simulink model "Adaptive_Distributed_Observer"  (R2016b)
settings: Solver=ode23t  StartTime=0.0  StopTime=5  RelTol=1e-3
values from neighbouring files (symbols this model uses):
  E = zeros(2,4)    [Init_ADO.m]
  F = -R    [Init_ADO.m]
  mu = 100    [Init_ADO.m]
  Mu_n = 100000    [Init_ADO.m]
  Mu_S = 10    [Init_ADO.m]
  P = [-2, -6]    [Init_ADO.m]
  R = [1 0 0 0]    [Init_ADO.m]
  S = [0 w1 0 0;-w1 0 0 0;0 0 0 w2;0 0 -w2 0]    [Init_ADO.m]
  S0 = zeros(4,4)    [Init_ADO.m]
  Z0 = ones(3*n,1)    [Init_ADO.m]
settings Model: Creator=Niels  LastModifiedBy=Niels
settings SolverCC: ZeroCrossAlgorithm=Adaptive

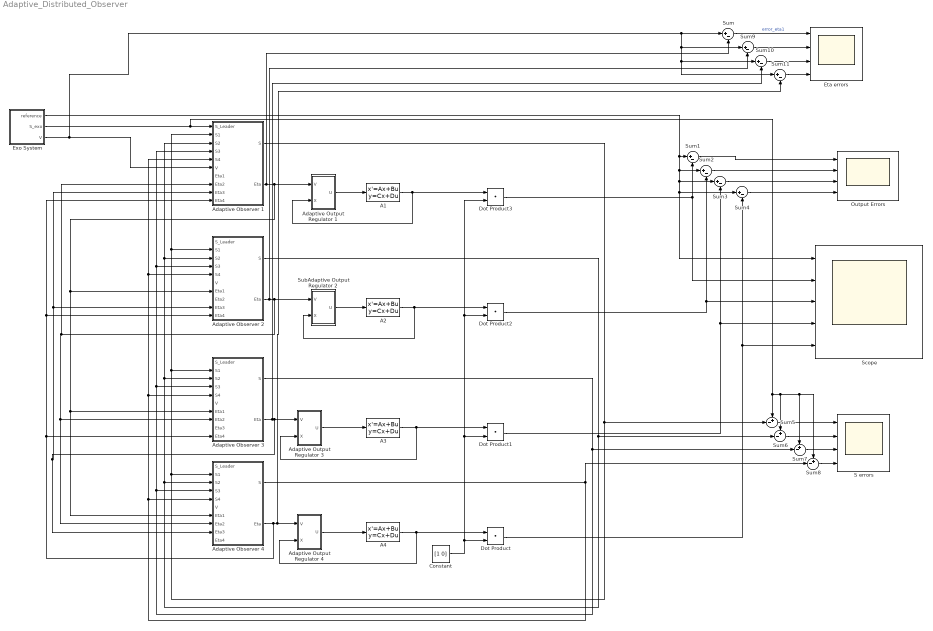
== system Adaptive_Distributed_Observer ==
  A1 : StateSpace  A=[-10 1;-24 0]  B=[2;3]  C=[1 0;0 1]  D=[0;0]  X0=0
  A2 : StateSpace  A=[-12 1;-11 0]  B=[2;1]  C=[1 0; 0 1]  D=[0;0]  X0=0
  A3 : StateSpace  A=[3 1;-1 0]  B=[1;1]  C=[1 0;0 1]  D=[0;0]  X0=0
  A4 : StateSpace  A=[2 1; -2 0]  B=[3;1]  C=[1 0;0 1]  D=[0 ;0]  X0=0
  Adaptive Observer 1 : Subsystem
  Adaptive Observer 2 : Subsystem
  Adaptive Observer 3 : Subsystem
  Adaptive Observer 4 : Subsystem
  Adaptive Output Regulator 1 : Subsystem
  Adaptive Output Regulator 3 : Subsystem
  Adaptive Output Regulator 4 : Subsystem
  Constant : Constant  Value=[1 0]
  Dot Product{,1..3} (4 alike) : DotProduct  InputSameDT=on  OutDataTypeStr=Inherit: Inherit via internal rule
  Eta errors : Scope  NumInputPorts=4
  Exo System : Subsystem
  Output Errors : Scope  NumInputPorts=4
  S errors : Scope  NumInputPorts=4
  Scope : Scope  NumInputPorts=5
  SubAdaptive Output Regulator 2 : Subsystem
  Sum{,1..4,9..11} (8 alike) : Sum  Inputs=|+-
  Sum{5..8} (4 alike) : Sum  Inputs=+-|
  wires:
  SubAdaptive Output Regulator 2/1(U) -> A2/1
  A4/1 -> Dot Product/1, Adaptive Output Regulator 4/2(X)
  A3/1 -> Dot Product1/1, Adaptive Output Regulator 3/2(X)
  Adaptive Observer 2/2(Eta) -> Sum9/2, SubAdaptive Output Regulator 2/1(V), Adaptive Observer 1/8(Eta2), Adaptive Observer 4/8(Eta2), Adaptive Observer 3/8(Eta2)
  Adaptive Observer 3/2(Eta) -> Adaptive Output Regulator 3/1(V), Adaptive Observer 1/9(Eta3), Adaptive Observer 2/9(Eta3), Adaptive Observer 4/9(Eta3), Sum10/2
  Adaptive Observer 4/2(Eta) -> Adaptive Output Regulator 4/1(V), Sum11/2, Adaptive Observer 1/10(Eta4), Adaptive Observer 2/10(Eta4), Adaptive Observer 3/10(Eta4)
  Exo System/3(V) -> Sum11/1, Sum10/1, Sum9/1, Sum/1, Adaptive Observer 1/6(V)
  Adaptive Observer 1/1(S) -> Sum5/2, Adaptive Observer 1/2("S1 "), Adaptive Observer 2/2("S1 "), Adaptive Observer 3/2("S1 "), Adaptive Observer 4/2("S1 ")
  Adaptive Observer 2/1(S) -> Adaptive Observer 1/3(S2), Adaptive Observer 2/3(S2), Adaptive Observer 3/3(S2), Adaptive Observer 4/3(S2), Sum6/2
  Adaptive Observer 3/1(S) -> Sum7/2, Adaptive Observer 1/4(S3), Adaptive Observer 2/4(S3), Adaptive Observer 3/4(S3), Adaptive Observer 4/4(S3)
  Adaptive Observer 4/1(S) -> Sum8/2, Adaptive Observer 1/5(S4), Adaptive Observer 2/5(S4), Adaptive Observer 3/5(S4), Adaptive Observer 4/5(S4)
  Adaptive Observer 1/2(Eta) -> Adaptive Output Regulator 1/1(V), Adaptive Observer 2/7(Eta1), Adaptive Observer 3/7(Eta1), Adaptive Observer 4/7(Eta1), Sum/2
  Exo System/1(reference) -> Scope/1, Sum4/1, Sum3/1, Sum2/1, Sum1/1
  A1/1 -> Dot Product3/1, Adaptive Output Regulator 1/2(X)
  Exo System/2("S_exo ") -> Sum8/1, Sum7/1, Sum6/1, Sum5/1, Adaptive Observer 1/1(S_Leader)
  Adaptive Output Regulator 1/1(U) -> A1/1
  Adaptive Output Regulator 3/1(U) -> A3/1
  Adaptive Output Regulator 4/1(U) -> A4/1
  Sum/1 -> Eta errors/1  "error_eta1"
  Sum1/1 -> Output Errors/1
  Sum2/1 -> Output Errors/2
  Sum3/1 -> Output Errors/3
  Sum4/1 -> Output Errors/4
  Sum8/1 -> S errors/4
  Sum7/1 -> S errors/3
  Sum5/1 -> S errors/1
  Sum6/1 -> S errors/2
  Sum9/1 -> Eta errors/2
  Sum10/1 -> Eta errors/3
  Sum11/1 -> Eta errors/4
  A2/1 -> Dot Product2/1, SubAdaptive Output Regulator 2/2(X)
  Dot Product/1 -> Scope/5, Sum4/2
  Dot Product1/1 -> Scope/4, Sum3/2
  Dot Product2/1 -> Scope/3, Sum2/2
  Dot Product3/1 -> Scope/2, Sum1/2
  Constant/1 -> Dot Product/2, Dot Product1/2, Dot Product2/2, Dot Product3/2

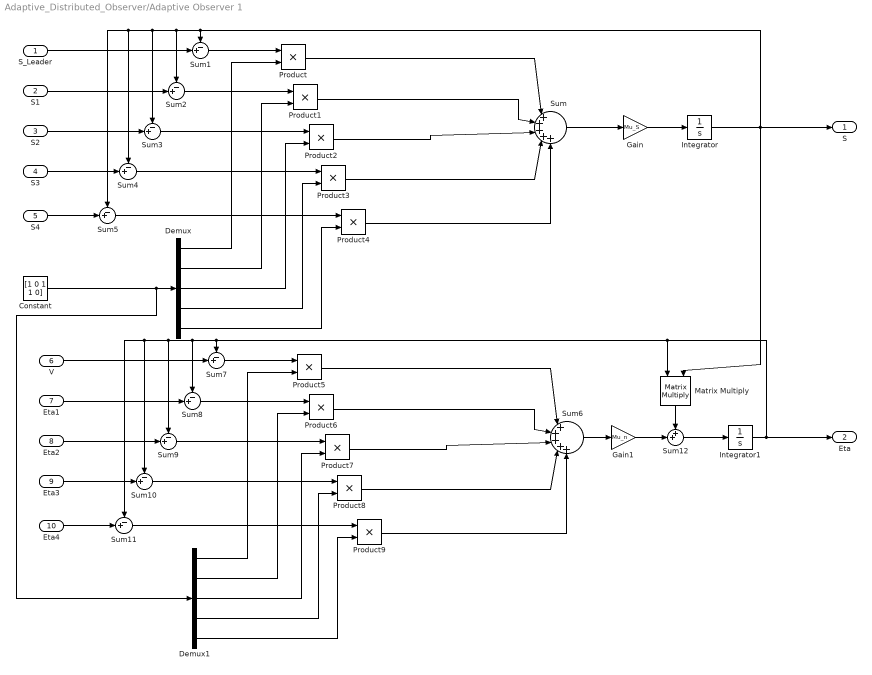
== system Adaptive_Distributed_Observer/Adaptive Observer 1 ==
  S_Leader : Inport
  "S1 " : Inport  Port=2
  S2 : Inport  Port=3
  S3 : Inport  Port=4
  S4 : Inport  Port=5
  V : Inport  Port=6
  Eta1 : Inport  Port=7
  Eta2 : Inport  Port=8
  Eta3 : Inport  Port=9
  Eta4 : Inport  Port=10
  Constant : Constant  Value=[1 0 1 1 0]
  Demux : Demux  Outputs=5
  Demux1 : Demux  Outputs=5
  Gain : Gain  Gain=Mu_S
  Gain1 : Gain  Gain=Mu_n
  Integrator : Integrator  InitialCondition=S0
  Integrator1 : Integrator
  Matrix Multiply : Product  Multiplication=Matrix(*)
  Product{,1..9} (10 alike) : Product
  Sum : Sum  Inputs=|+++++
  Sum{1..5,7..11} (10 alike) : Sum  Inputs=-+|
  Sum12 : Sum  Inputs=++|
  Sum6 : Sum  Inputs=|+++++
  S : Outport
  Eta : Outport  Port=2
  wires:
  Demux/1 -> Product/2
  Demux/2 -> Product1/2
  Demux/3 -> Product2/2
  Demux/4 -> Product3/2
  Demux/5 -> Product4/2
  Product2/1 -> Sum/3
  Product1/1 -> Sum/2
  Product/1 -> Sum/1
  Product4/1 -> Sum/5
  Product3/1 -> Sum/4
  Sum/1 -> Gain/1
  Gain/1 -> Integrator/1
  Sum1/1 -> Product/1
  S_Leader/1 -> Sum1/2
  "S1 "/1 -> Sum2/2
  Sum2/1 -> Product1/1
  S2/1 -> Sum3/2
  Sum3/1 -> Product2/1
  S3/1 -> Sum4/2
  Sum4/1 -> Product3/1
  S4/1 -> Sum5/2
  Sum5/1 -> Product4/1
  Integrator/1 -> Matrix Multiply/2, Sum3/1, Sum4/1, Sum5/1, Sum2/1, Sum1/1, S/1
  Demux1/1 -> Product5/2
  Demux1/2 -> Product6/2
  Demux1/3 -> Product7/2
  Demux1/4 -> Product8/2
  Demux1/5 -> Product9/2
  Product7/1 -> Sum6/3
  Product6/1 -> Sum6/2
  Product5/1 -> Sum6/1
  Product9/1 -> Sum6/5
  Product8/1 -> Sum6/4
  Sum6/1 -> Gain1/1
  Sum7/1 -> Product5/1
  V/1 -> Sum7/2
  Eta1/1 -> Sum8/2
  Sum8/1 -> Product6/1
  Eta2/1 -> Sum9/2
  Sum9/1 -> Product7/1
  Eta3/1 -> Sum10/2
  Sum10/1 -> Product8/1
  Sum11/1 -> Product9/1
  Integrator1/1 -> Eta/1, Matrix Multiply/1, Sum9/1, Sum10/1, Sum11/1, Sum8/1, Sum7/1
  Constant/1 -> Demux1/1, Demux/1
  Eta4/1 -> Sum11/2
  Sum12/1 -> Integrator1/1
  Gain1/1 -> Sum12/2
  Matrix Multiply/1 -> Sum12/1

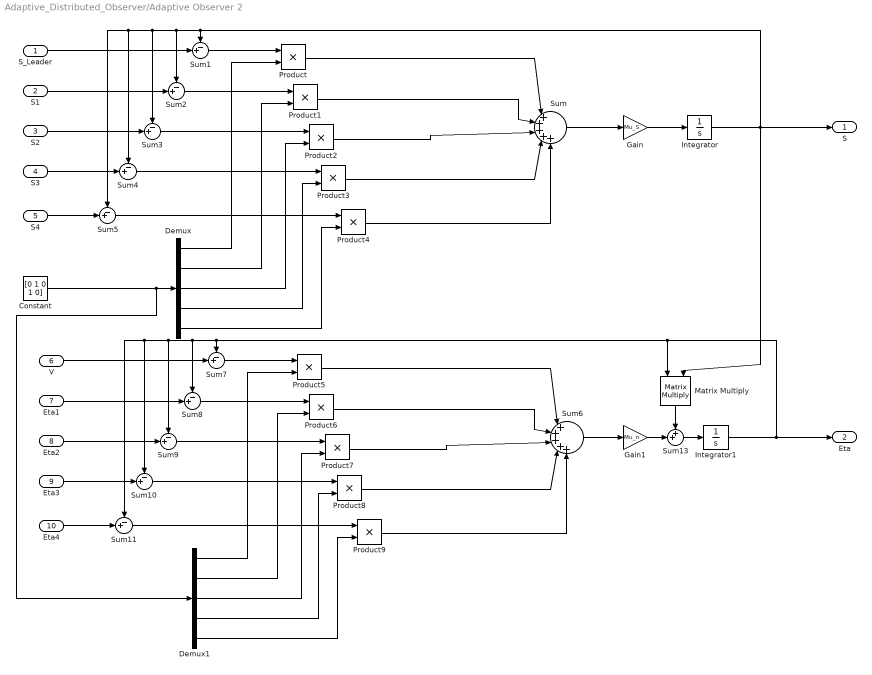
== system Adaptive_Distributed_Observer/Adaptive Observer 2 ==
  S_Leader : Inport
  "S1 " : Inport  Port=2
  S2 : Inport  Port=3
  S3 : Inport  Port=4
  S4 : Inport  Port=5
  V : Inport  Port=6
  Eta1 : Inport  Port=7
  Eta2 : Inport  Port=8
  Eta3 : Inport  Port=9
  Eta4 : Inport  Port=10
  Constant : Constant  Value=[0 1 0 1 0]
  Demux : Demux  Outputs=5
  Demux1 : Demux  Outputs=5
  Gain : Gain  Gain=Mu_S
  Gain1 : Gain  Gain=Mu_n
  Integrator : Integrator  InitialCondition=S0
  Integrator1 : Integrator
  Matrix Multiply : Product  Multiplication=Matrix(*)
  Product{,1..9} (10 alike) : Product
  Sum : Sum  Inputs=|+++++
  Sum{1..5,7..11} (10 alike) : Sum  Inputs=-+|
  Sum13 : Sum  Inputs=++|
  Sum6 : Sum  Inputs=|+++++
  S : Outport
  Eta : Outport  Port=2
  wires:
  Demux/1 -> Product/2
  Demux/2 -> Product1/2
  Demux/3 -> Product2/2
  Demux/4 -> Product3/2
  Demux/5 -> Product4/2
  Product2/1 -> Sum/3
  Product1/1 -> Sum/2
  Product/1 -> Sum/1
  Product4/1 -> Sum/5
  Product3/1 -> Sum/4
  Sum/1 -> Gain/1
  Gain/1 -> Integrator/1
  Sum1/1 -> Product/1
  S_Leader/1 -> Sum1/2
  "S1 "/1 -> Sum2/2
  Sum2/1 -> Product1/1
  S2/1 -> Sum3/2
  Sum3/1 -> Product2/1
  S3/1 -> Sum4/2
  Sum4/1 -> Product3/1
  S4/1 -> Sum5/2
  Sum5/1 -> Product4/1
  Demux1/1 -> Product5/2
  Demux1/2 -> Product6/2
  Demux1/3 -> Product7/2
  Demux1/4 -> Product8/2
  Demux1/5 -> Product9/2
  Product7/1 -> Sum6/3
  Product6/1 -> Sum6/2
  Product5/1 -> Sum6/1
  Product9/1 -> Sum6/5
  Product8/1 -> Sum6/4
  Sum6/1 -> Gain1/1
  Sum7/1 -> Product5/1
  V/1 -> Sum7/2
  Eta1/1 -> Sum8/2
  Sum8/1 -> Product6/1
  Eta2/1 -> Sum9/2
  Sum9/1 -> Product7/1
  Eta3/1 -> Sum10/2
  Sum10/1 -> Product8/1
  Sum11/1 -> Product9/1
  Constant/1 -> Demux1/1, Demux/1
  Eta4/1 -> Sum11/2
  Integrator/1 -> Matrix Multiply/2, Sum3/1, Sum4/1, Sum5/1, Sum2/1, Sum1/1, S/1
  Integrator1/1 -> Eta/1, Matrix Multiply/1, Sum9/1, Sum10/1, Sum11/1, Sum8/1, Sum7/1
  Gain1/1 -> Sum13/2
  Sum13/1 -> Integrator1/1
  Matrix Multiply/1 -> Sum13/1

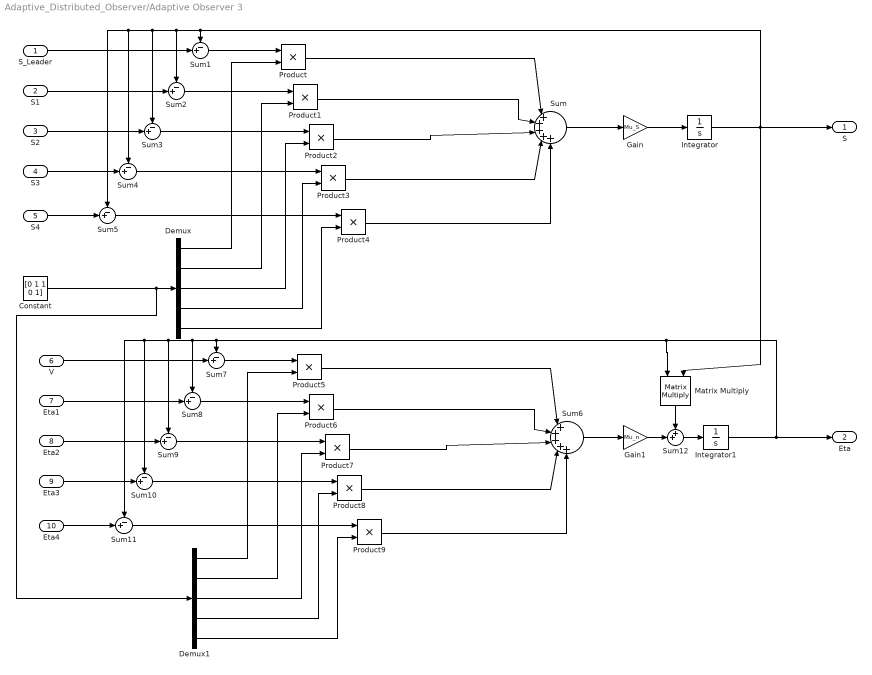
== system Adaptive_Distributed_Observer/Adaptive Observer 3 ==
  S_Leader : Inport
  "S1 " : Inport  Port=2
  S2 : Inport  Port=3
  S3 : Inport  Port=4
  S4 : Inport  Port=5
  V : Inport  Port=6
  Eta1 : Inport  Port=7
  Eta2 : Inport  Port=8
  Eta3 : Inport  Port=9
  Eta4 : Inport  Port=10
  Constant : Constant  Value=[0 1 1 0 1]
  Demux : Demux  Outputs=5
  Demux1 : Demux  Outputs=5
  Gain : Gain  Gain=Mu_S
  Gain1 : Gain  Gain=Mu_n
  Integrator : Integrator  InitialCondition=S0
  Integrator1 : Integrator
  Matrix Multiply : Product  Multiplication=Matrix(*)
  Product{,1..9} (10 alike) : Product
  Sum : Sum  Inputs=|+++++
  Sum{1..5,7..11} (10 alike) : Sum  Inputs=-+|
  Sum12 : Sum  Inputs=++|
  Sum6 : Sum  Inputs=|+++++
  S : Outport
  Eta : Outport  Port=2
  wires:
  Demux/1 -> Product/2
  Demux/2 -> Product1/2
  Demux/3 -> Product2/2
  Demux/4 -> Product3/2
  Demux/5 -> Product4/2
  Product2/1 -> Sum/3
  Product1/1 -> Sum/2
  Product/1 -> Sum/1
  Product4/1 -> Sum/5
  Product3/1 -> Sum/4
  Sum/1 -> Gain/1
  Gain/1 -> Integrator/1
  Sum1/1 -> Product/1
  S_Leader/1 -> Sum1/2
  "S1 "/1 -> Sum2/2
  Sum2/1 -> Product1/1
  S2/1 -> Sum3/2
  Sum3/1 -> Product2/1
  S3/1 -> Sum4/2
  Sum4/1 -> Product3/1
  S4/1 -> Sum5/2
  Sum5/1 -> Product4/1
  Demux1/1 -> Product5/2
  Demux1/2 -> Product6/2
  Demux1/3 -> Product7/2
  Demux1/4 -> Product8/2
  Demux1/5 -> Product9/2
  Product7/1 -> Sum6/3
  Product6/1 -> Sum6/2
  Product5/1 -> Sum6/1
  Product9/1 -> Sum6/5
  Product8/1 -> Sum6/4
  Sum6/1 -> Gain1/1
  Sum7/1 -> Product5/1
  V/1 -> Sum7/2
  Eta1/1 -> Sum8/2
  Sum8/1 -> Product6/1
  Eta2/1 -> Sum9/2
  Sum9/1 -> Product7/1
  Eta3/1 -> Sum10/2
  Sum10/1 -> Product8/1
  Sum11/1 -> Product9/1
  Constant/1 -> Demux1/1, Demux/1
  Eta4/1 -> Sum11/2
  Integrator/1 -> Matrix Multiply/2, Sum3/1, Sum4/1, Sum5/1, Sum2/1, Sum1/1, S/1
  Integrator1/1 -> Eta/1, Matrix Multiply/1, Sum9/1, Sum10/1, Sum11/1, Sum8/1, Sum7/1
  Gain1/1 -> Sum12/2
  Sum12/1 -> Integrator1/1
  Matrix Multiply/1 -> Sum12/1

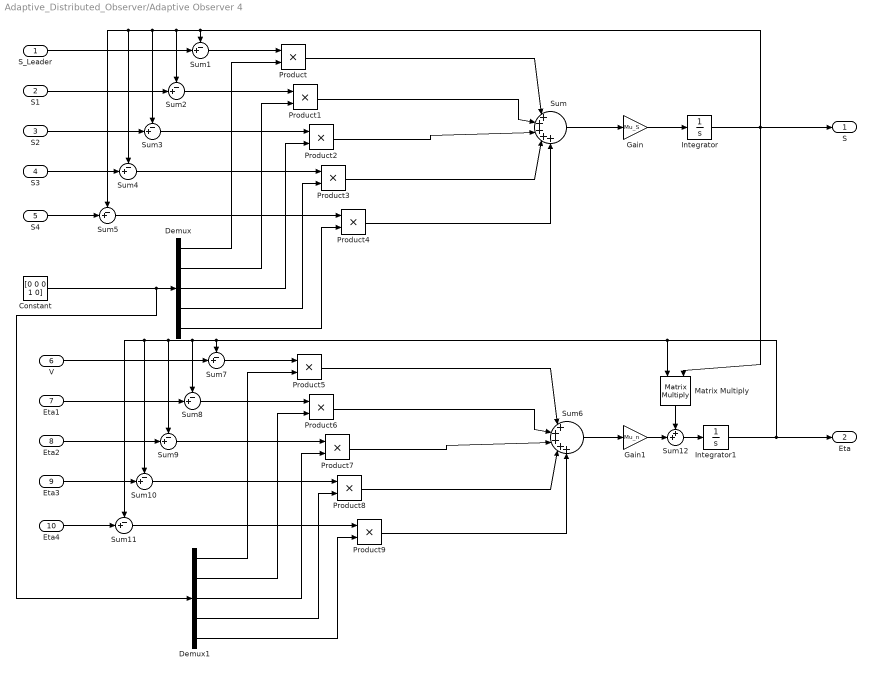
== system Adaptive_Distributed_Observer/Adaptive Observer 4 ==
  S_Leader : Inport
  "S1 " : Inport  Port=2
  S2 : Inport  Port=3
  S3 : Inport  Port=4
  S4 : Inport  Port=5
  V : Inport  Port=6
  Eta1 : Inport  Port=7
  Eta2 : Inport  Port=8
  Eta3 : Inport  Port=9
  Eta4 : Inport  Port=10
  Constant : Constant  Value=[0 0 0 1 0]
  Demux : Demux  Outputs=5
  Demux1 : Demux  Outputs=5
  Gain : Gain  Gain=Mu_S
  Gain1 : Gain  Gain=Mu_n
  Integrator : Integrator  InitialCondition=S0
  Integrator1 : Integrator
  Matrix Multiply : Product  Multiplication=Matrix(*)
  Product{,1..9} (10 alike) : Product
  Sum : Sum  Inputs=|+++++
  Sum{1..5,7..11} (10 alike) : Sum  Inputs=-+|
  Sum12 : Sum  Inputs=++|
  Sum6 : Sum  Inputs=|+++++
  S : Outport
  Eta : Outport  Port=2
  wires:
  Demux/1 -> Product/2
  Demux/2 -> Product1/2
  Demux/3 -> Product2/2
  Demux/4 -> Product3/2
  Demux/5 -> Product4/2
  Product2/1 -> Sum/3
  Product1/1 -> Sum/2
  Product/1 -> Sum/1
  Product4/1 -> Sum/5
  Product3/1 -> Sum/4
  Sum/1 -> Gain/1
  Gain/1 -> Integrator/1
  Sum1/1 -> Product/1
  S_Leader/1 -> Sum1/2
  "S1 "/1 -> Sum2/2
  Sum2/1 -> Product1/1
  S2/1 -> Sum3/2
  Sum3/1 -> Product2/1
  S3/1 -> Sum4/2
  Sum4/1 -> Product3/1
  S4/1 -> Sum5/2
  Sum5/1 -> Product4/1
  Demux1/1 -> Product5/2
  Demux1/2 -> Product6/2
  Demux1/3 -> Product7/2
  Demux1/4 -> Product8/2
  Demux1/5 -> Product9/2
  Product7/1 -> Sum6/3
  Product6/1 -> Sum6/2
  Product5/1 -> Sum6/1
  Product9/1 -> Sum6/5
  Product8/1 -> Sum6/4
  Sum6/1 -> Gain1/1
  Sum7/1 -> Product5/1
  V/1 -> Sum7/2
  Eta1/1 -> Sum8/2
  Sum8/1 -> Product6/1
  Eta2/1 -> Sum9/2
  Sum9/1 -> Product7/1
  Eta3/1 -> Sum10/2
  Sum10/1 -> Product8/1
  Sum11/1 -> Product9/1
  Constant/1 -> Demux1/1, Demux/1
  Eta4/1 -> Sum11/2
  Integrator/1 -> Matrix Multiply/2, Sum3/1, Sum4/1, Sum5/1, Sum2/1, Sum1/1, S/1
  Integrator1/1 -> Eta/1, Matrix Multiply/1, Sum9/1, Sum10/1, Sum11/1, Sum8/1, Sum7/1
  Gain1/1 -> Sum12/2
  Sum12/1 -> Integrator1/1
  Matrix Multiply/1 -> Sum12/1

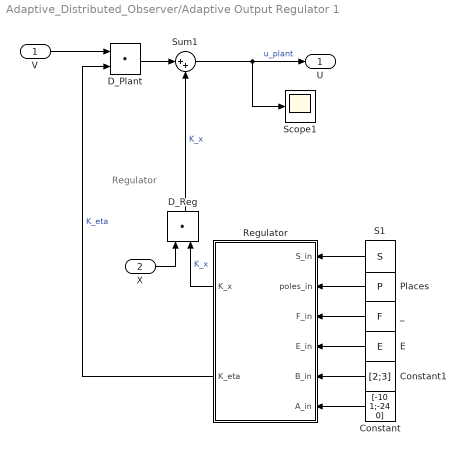
== system Adaptive_Distributed_Observer/Adaptive Output Regulator 1 ==
  note: Regulator
  V : Inport
  X : Inport  Port=2
  Constant : Constant  Value=[-10 1;-24 0]
  Constant1 : Constant  Value=[2;3]
  D_Plant : DotProduct  InputSameDT=on  OutDataTypeStr=Inherit: Inherit via internal rule
  "D_Reg " : DotProduct  InputSameDT=on  OutDataTypeStr=Inherit: Inherit via internal rule
  E : Constant  Value=E
  Places : Constant  Value=P  VectorParams1D=off
  Regulator : Subsystem
  S1 : Constant  Value=S
  Scope1 : Scope
  Sum1 : Sum  Inputs=|++
  _ : Constant  Value=F  VectorParams1D=off
  U : Outport
  wires:
  V/1 -> D_Plant/1
  S1/1 -> Regulator/1(S_in)
  D_Plant/1 -> Sum1/1
  Regulator/1(K_x) -> "D_Reg "/2  "K_x"
  E/1 -> Regulator/4(E_in)
  _/1 -> Regulator/3(F_in)
  Regulator/2(K_eta) -> D_Plant/2  "K_eta"
  "D_Reg "/1 -> Sum1/2  "K_x"
  Places/1 -> Regulator/2(poles_in)
  Sum1/1 -> U/1, Scope1/1  "u_plant"
  X/1 -> "D_Reg "/1
  Constant/1 -> Regulator/6(A_in)
  Constant1/1 -> Regulator/5(B_in)

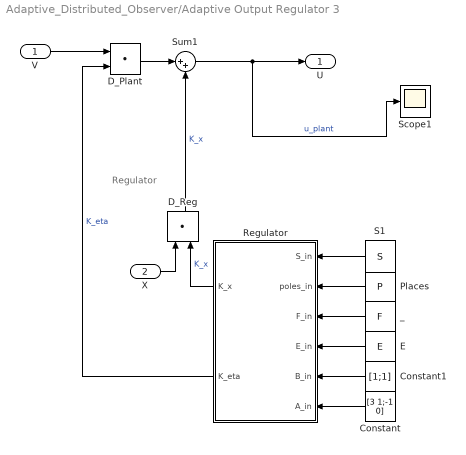
== system Adaptive_Distributed_Observer/Adaptive Output Regulator 3 ==
  note: Regulator
  V : Inport
  X : Inport  Port=2
  Constant : Constant  Value=[3 1;-1 0]
  Constant1 : Constant  Value=[1;1]
  D_Plant : DotProduct  InputSameDT=on  OutDataTypeStr=Inherit: Inherit via internal rule
  "D_Reg " : DotProduct  InputSameDT=on  OutDataTypeStr=Inherit: Inherit via internal rule
  E : Constant  Value=E
  Places : Constant  Value=P  VectorParams1D=off
  Regulator : Subsystem
  S1 : Constant  Value=S
  Scope1 : Scope
  Sum1 : Sum  Inputs=|++
  _ : Constant  Value=F  VectorParams1D=off
  U : Outport
  wires:
  V/1 -> D_Plant/1
  S1/1 -> Regulator/1(S_in)
  D_Plant/1 -> Sum1/1
  Regulator/1(K_x) -> "D_Reg "/2  "K_x"
  E/1 -> Regulator/4(E_in)
  _/1 -> Regulator/3(F_in)
  Regulator/2(K_eta) -> D_Plant/2  "K_eta"
  "D_Reg "/1 -> Sum1/2  "K_x"
  Places/1 -> Regulator/2(poles_in)
  Sum1/1 -> U/1, Scope1/1  "u_plant"
  X/1 -> "D_Reg "/1
  Constant/1 -> Regulator/6(A_in)
  Constant1/1 -> Regulator/5(B_in)

== system Adaptive_Distributed_Observer/Adaptive Output Regulator 4 ==
  note: Regulator
  V : Inport
  X : Inport  Port=2
  Constant : Constant  Value=[2 1;-2 0]
  Constant1 : Constant  Value=[3;1]
  D_Plant : DotProduct  InputSameDT=on  OutDataTypeStr=Inherit: Inherit via internal rule
  "D_Reg " : DotProduct  InputSameDT=on  OutDataTypeStr=Inherit: Inherit via internal rule
  E : Constant  Value=E
  Places : Constant  Value=P  VectorParams1D=off
  Regulator : Subsystem
  S1 : Constant  Value=S
  Sum1 : Sum  Inputs=|++
  _ : Constant  Value=F  VectorParams1D=off
  U : Outport
  wires:
  V/1 -> D_Plant/1
  S1/1 -> Regulator/1(S_in)
  D_Plant/1 -> Sum1/1
  Regulator/1(K_x) -> "D_Reg "/2  "K_x"
  E/1 -> Regulator/4(E_in)
  _/1 -> Regulator/3(F_in)
  Regulator/2(K_eta) -> D_Plant/2  "K_eta"
  "D_Reg "/1 -> Sum1/2  "K_x"
  Places/1 -> Regulator/2(poles_in)
  Sum1/1 -> U/1  "u_plant"
  Constant/1 -> Regulator/6(A_in)
  Constant1/1 -> Regulator/5(B_in)
  X/1 -> "D_Reg "/1

== system Adaptive_Distributed_Observer/Exo System ==
  Dot Product : DotProduct  InputSameDT=on  OutDataTypeStr=Inherit: Inherit via internal rule
  I_exo : Integrator  InitialCondition=[1;0;1;0]
  Matrix Multiply : Product  Multiplication=Matrix(*)
  "R " : Constant  Value=R
  S : Constant  Value=S
  reference : Outport
  "S_exo " : Outport  Port=2
  V : Outport  Port=3
  wires:
  I_exo/1 -> Matrix Multiply/2, Dot Product/1, V/1
  "R "/1 -> Dot Product/2
  Dot Product/1 -> reference/1
  Matrix Multiply/1 -> I_exo/1
  S/1 -> "S_exo "/1, Matrix Multiply/1

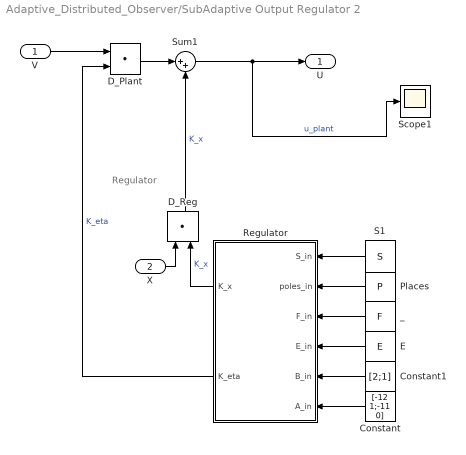
== system Adaptive_Distributed_Observer/SubAdaptive Output Regulator 2 ==
  note: Regulator
  V : Inport
  X : Inport  Port=2
  Constant : Constant  Value=[-12 1;-11 0]
  Constant1 : Constant  Value=[2;1]
  D_Plant : DotProduct  InputSameDT=on  OutDataTypeStr=Inherit: Inherit via internal rule
  "D_Reg " : DotProduct  InputSameDT=on  OutDataTypeStr=Inherit: Inherit via internal rule
  E : Constant  Value=E
  Places : Constant  Value=P  VectorParams1D=off
  Regulator : Subsystem
  S1 : Constant  Value=S
  Scope1 : Scope
  Sum1 : Sum  Inputs=|++
  _ : Constant  Value=F  VectorParams1D=off
  U : Outport
  wires:
  V/1 -> D_Plant/1
  S1/1 -> Regulator/1(S_in)
  D_Plant/1 -> Sum1/1
  Regulator/1(K_x) -> "D_Reg "/2  "K_x"
  E/1 -> Regulator/4(E_in)
  _/1 -> Regulator/3(F_in)
  Regulator/2(K_eta) -> D_Plant/2  "K_eta"
  "D_Reg "/1 -> Sum1/2  "K_x"
  Places/1 -> Regulator/2(poles_in)
  Sum1/1 -> U/1, Scope1/1  "u_plant"
  X/1 -> "D_Reg "/1
  Constant/1 -> Regulator/6(A_in)
  Constant1/1 -> Regulator/5(B_in)

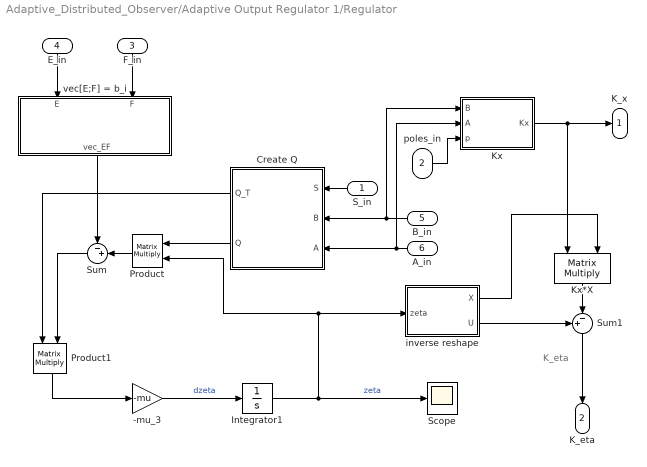
== system Adaptive_Distributed_Observer/Adaptive Output Regulator 1/Regulator ==
  note: K_eta
  S_in : Inport
  poles_in : Inport  Port=2
  F_in : Inport  Port=3
  E_in : Inport  Port=4
  B_in : Inport  Port=5
  A_in : Inport  Port=6
  -mu_3 : Gain  Gain=-mu
  Create Q : MATLAB Function  TreatAsAtomicUnit=on
  Integrator1 : Integrator  InitialCondition=Z0
  Kx : MATLAB Function  TreatAsAtomicUnit=on
  Kx*X : Product  Inputs=**  Multiplication=Matrix(*)
  Product : Product  Multiplication=Matrix(*)
  Product1 : Product  Multiplication=Matrix(*)
  Scope : Scope
  Sum : Sum  Inputs=-+|
  Sum1 : Sum  Inputs=+-|
  inverse reshape : MATLAB Function  TreatAsAtomicUnit=on
  "vec[E;F] = b_i   " : MATLAB Function  TreatAsAtomicUnit=on
  K_x : Outport
  K_eta : Outport  Port=2
  wires:
  Product/1 -> Sum/2
  "vec[E;F] = b_i   "/1(vec_EF) -> Sum/1
  E_in/1 -> "vec[E;F] = b_i   "/1(E)
  B_in/1 -> Create Q/2(B), Kx/1(B)
  A_in/1 -> Kx/2(A), Create Q/3(A)
  S_in/1 -> Create Q/1(S)
  Kx/1(Kx) -> K_x/1, Kx*X/1
  -mu_3/1 -> Integrator1/1  "dzeta"
  Integrator1/1 -> Product/2, inverse reshape/1(zeta), Scope/1  "zeta"
  poles_in/1 -> Kx/3(p)
  Kx*X/1 -> Sum1/2
  Create Q/1(Q_T) -> Product1/1
  Sum/1 -> Product1/2
  Sum1/1 -> K_eta/1
  Product1/1 -> -mu_3/1
  Create Q/2(Q) -> Product/1
  F_in/1 -> "vec[E;F] = b_i   "/2(F)
  inverse reshape/2(U) -> Sum1/1
  inverse reshape/1(X) -> Kx*X/2

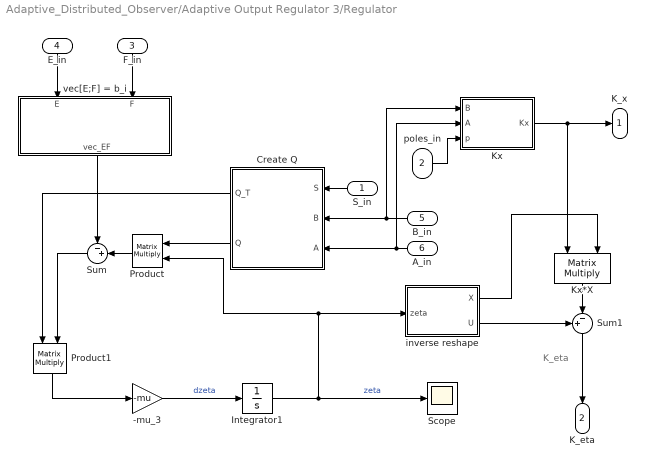
== system Adaptive_Distributed_Observer/Adaptive Output Regulator 3/Regulator ==
  note: K_eta
  S_in : Inport
  poles_in : Inport  Port=2
  F_in : Inport  Port=3
  E_in : Inport  Port=4
  B_in : Inport  Port=5
  A_in : Inport  Port=6
  -mu_3 : Gain  Gain=-mu
  Create Q : MATLAB Function  TreatAsAtomicUnit=on
  Integrator1 : Integrator  InitialCondition=Z0
  Kx : MATLAB Function  TreatAsAtomicUnit=on
  Kx*X : Product  Inputs=**  Multiplication=Matrix(*)
  Product : Product  Multiplication=Matrix(*)
  Product1 : Product  Multiplication=Matrix(*)
  Scope : Scope
  Sum : Sum  Inputs=-+|
  Sum1 : Sum  Inputs=+-|
  inverse reshape : MATLAB Function  TreatAsAtomicUnit=on
  "vec[E;F] = b_i   " : MATLAB Function  TreatAsAtomicUnit=on
  K_x : Outport
  K_eta : Outport  Port=2
  wires:
  Product/1 -> Sum/2
  "vec[E;F] = b_i   "/1(vec_EF) -> Sum/1
  E_in/1 -> "vec[E;F] = b_i   "/1(E)
  B_in/1 -> Create Q/2(B), Kx/1(B)
  A_in/1 -> Kx/2(A), Create Q/3(A)
  S_in/1 -> Create Q/1(S)
  Kx/1(Kx) -> K_x/1, Kx*X/1
  -mu_3/1 -> Integrator1/1  "dzeta"
  Integrator1/1 -> Product/2, inverse reshape/1(zeta), Scope/1  "zeta"
  poles_in/1 -> Kx/3(p)
  Kx*X/1 -> Sum1/2
  Create Q/1(Q_T) -> Product1/1
  Sum/1 -> Product1/2
  Sum1/1 -> K_eta/1
  Product1/1 -> -mu_3/1
  Create Q/2(Q) -> Product/1
  F_in/1 -> "vec[E;F] = b_i   "/2(F)
  inverse reshape/2(U) -> Sum1/1
  inverse reshape/1(X) -> Kx*X/2

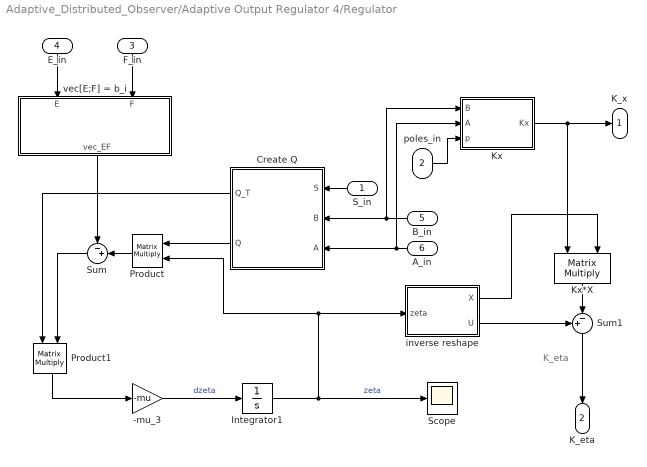
== system Adaptive_Distributed_Observer/Adaptive Output Regulator 4/Regulator ==
  note: K_eta
  S_in : Inport
  poles_in : Inport  Port=2
  F_in : Inport  Port=3
  E_in : Inport  Port=4
  B_in : Inport  Port=5
  A_in : Inport  Port=6
  -mu_3 : Gain  Gain=-mu
  Create Q : MATLAB Function  TreatAsAtomicUnit=on
  Integrator1 : Integrator  InitialCondition=Z0
  Kx : MATLAB Function  TreatAsAtomicUnit=on
  Kx*X : Product  Inputs=**  Multiplication=Matrix(*)
  Product : Product  Multiplication=Matrix(*)
  Product1 : Product  Multiplication=Matrix(*)
  Scope : Scope
  Sum : Sum  Inputs=-+|
  Sum1 : Sum  Inputs=+-|
  inverse reshape : MATLAB Function  TreatAsAtomicUnit=on
  "vec[E;F] = b_i   " : MATLAB Function  TreatAsAtomicUnit=on
  K_x : Outport
  K_eta : Outport  Port=2
  wires:
  Product/1 -> Sum/2
  "vec[E;F] = b_i   "/1(vec_EF) -> Sum/1
  E_in/1 -> "vec[E;F] = b_i   "/1(E)
  B_in/1 -> Create Q/2(B), Kx/1(B)
  A_in/1 -> Kx/2(A), Create Q/3(A)
  S_in/1 -> Create Q/1(S)
  Kx/1(Kx) -> K_x/1, Kx*X/1
  -mu_3/1 -> Integrator1/1  "dzeta"
  Integrator1/1 -> Product/2, inverse reshape/1(zeta), Scope/1  "zeta"
  poles_in/1 -> Kx/3(p)
  Kx*X/1 -> Sum1/2
  Create Q/1(Q_T) -> Product1/1
  Sum/1 -> Product1/2
  Sum1/1 -> K_eta/1
  Product1/1 -> -mu_3/1
  Create Q/2(Q) -> Product/1
  F_in/1 -> "vec[E;F] = b_i   "/2(F)
  inverse reshape/2(U) -> Sum1/1
  inverse reshape/1(X) -> Kx*X/2

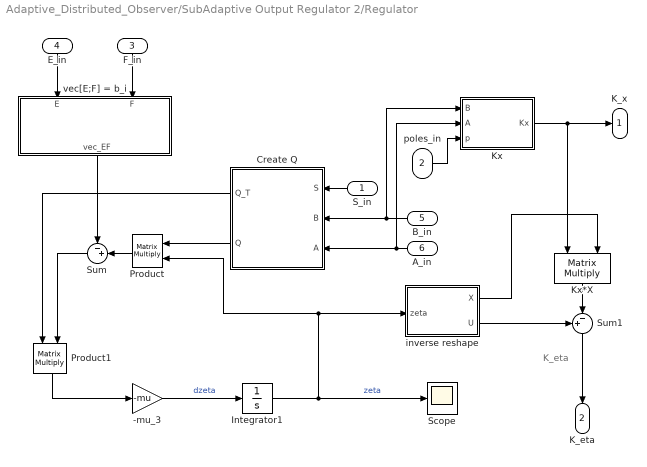
== system Adaptive_Distributed_Observer/SubAdaptive Output Regulator 2/Regulator ==
  note: K_eta
  S_in : Inport
  poles_in : Inport  Port=2
  F_in : Inport  Port=3
  E_in : Inport  Port=4
  B_in : Inport  Port=5
  A_in : Inport  Port=6
  -mu_3 : Gain  Gain=-mu
  Create Q : MATLAB Function  TreatAsAtomicUnit=on
  Integrator1 : Integrator  InitialCondition=Z0
  Kx : MATLAB Function  TreatAsAtomicUnit=on
  Kx*X : Product  Inputs=**  Multiplication=Matrix(*)
  Product : Product  Multiplication=Matrix(*)
  Product1 : Product  Multiplication=Matrix(*)
  Scope : Scope
  Sum : Sum  Inputs=-+|
  Sum1 : Sum  Inputs=+-|
  inverse reshape : MATLAB Function  TreatAsAtomicUnit=on
  "vec[E;F] = b_i   " : MATLAB Function  TreatAsAtomicUnit=on
  K_x : Outport
  K_eta : Outport  Port=2
  wires:
  Product/1 -> Sum/2
  "vec[E;F] = b_i   "/1(vec_EF) -> Sum/1
  E_in/1 -> "vec[E;F] = b_i   "/1(E)
  B_in/1 -> Create Q/2(B), Kx/1(B)
  A_in/1 -> Kx/2(A), Create Q/3(A)
  S_in/1 -> Create Q/1(S)
  Kx/1(Kx) -> K_x/1, Kx*X/1
  -mu_3/1 -> Integrator1/1  "dzeta"
  Integrator1/1 -> Product/2, inverse reshape/1(zeta), Scope/1  "zeta"
  poles_in/1 -> Kx/3(p)
  Kx*X/1 -> Sum1/2
  Create Q/1(Q_T) -> Product1/1
  Sum/1 -> Product1/2
  Sum1/1 -> K_eta/1
  Product1/1 -> -mu_3/1
  Create Q/2(Q) -> Product/1
  F_in/1 -> "vec[E;F] = b_i   "/2(F)
  inverse reshape/2(U) -> Sum1/1
  inverse reshape/1(X) -> Kx*X/2

== matlab function Adaptive_Distributed_Observer/Adaptive Output Regulator 1/Regulator/Create Q ==
  data: Q_T output size=[3*n,3*n]; Q output size=[3*n,3*n]; S input; B input; A input
function [Q_T,Q]= fcn(S,B,A)
[Sc,Sr]=size(S);
I_ni = [eye(2) zeros(2,1);zeros(1,3)];
I_q = eye(Sc);
sysmatrix = [A B;1 0 0];

Q = kron(S.',I_ni)-kron(I_q,sysmatrix);
Q_T = Q.';
end

== matlab function Adaptive_Distributed_Observer/Adaptive Output Regulator 1/Regulator/Kx ==
  data: B input; A input; Kx output; p input
function Kx = fcn(B,A,p)

coder.extrinsic('place')
Kx = zeros(1,2);
Kx = place(A,-B,p);

== matlab function Adaptive_Distributed_Observer/SubAdaptive Output Regulator 2/Regulator/Create Q ==
  data: Q_T output size=[3*n,3*n]; Q output size=[3*n,3*n]; S input; B input; A input
function [Q_T,Q]= fcn(S,B,A)
[Sc,Sr]=size(S);
I_ni = [eye(2) zeros(2,1);zeros(1,3)];
I_q = eye(Sc);
sysmatrix = [A B;1 0 0];

Q = kron(S.',I_ni)-kron(I_q,sysmatrix);
Q_T = Q.';
end

== matlab function Adaptive_Distributed_Observer/SubAdaptive Output Regulator 2/Regulator/Kx ==
  data: B input; A input; Kx output; p input
function Kx = fcn(B,A,p)

coder.extrinsic('place')
Kx = zeros(1,2);
Kx = place(A,-B,p);

== matlab function Adaptive_Distributed_Observer/SubAdaptive Output Regulator 2/Regulator/inverse reshape ==
  data: zeta input; X output; U output
function [X,U] = fcn(zeta)
n = 4;
tmp = reshape(zeta,3,n);
X = tmp(1:2,1:n);
U = tmp(3,:);
end

== matlab function Adaptive_Distributed_Observer/SubAdaptive Output Regulator 2/Regulator/vec[E;F] = b_i    ==
  data: E input; vec_EF output; F input
function vec_EF = fcn(E,F)
[Ec,Er] = size(E);
[Fc,Fr] = size(F);
vec_EF = reshape([E;F],Ec*Er+Fc*Fr,1);
end

== matlab function Adaptive_Distributed_Observer/Adaptive Output Regulator 1/Regulator/inverse reshape ==
  data: zeta input; X output; U output
function [X,U] = fcn(zeta)
n = 4;
tmp = reshape(zeta,3,n);
X = tmp(1:2,1:n);
U = tmp(3,:);
end

== matlab function Adaptive_Distributed_Observer/Adaptive Output Regulator 1/Regulator/vec[E;F] = b_i    ==
  data: E input; vec_EF output; F input
function vec_EF = fcn(E,F)
[Ec,Er] = size(E);
[Fc,Fr] = size(F);
vec_EF = reshape([E;F],Ec*Er+Fc*Fr,1);
end

== matlab function Adaptive_Distributed_Observer/Adaptive Output Regulator 3/Regulator/Create Q ==
  data: Q_T output size=[3*n,3*n]; Q output size=[3*n,3*n]; S input; B input; A input
function [Q_T,Q]= fcn(S,B,A)
[Sc,Sr]=size(S);
I_ni = [eye(2) zeros(2,1);zeros(1,3)];
I_q = eye(Sc);
sysmatrix = [A B;1 0 0];

Q = kron(S.',I_ni)-kron(I_q,sysmatrix);
Q_T = Q.';
end

== matlab function Adaptive_Distributed_Observer/Adaptive Output Regulator 3/Regulator/Kx ==
  data: B input; A input; Kx output; p input
function Kx = fcn(B,A,p)

coder.extrinsic('place')
Kx = zeros(1,2);
Kx = place(A,-B,p);

== matlab function Adaptive_Distributed_Observer/Adaptive Output Regulator 3/Regulator/inverse reshape ==
  data: zeta input; X output; U output
function [X,U] = fcn(zeta)
n = 4;
tmp = reshape(zeta,3,n);
X = tmp(1:2,1:n);
U = tmp(3,:);
end

== matlab function Adaptive_Distributed_Observer/Adaptive Output Regulator 3/Regulator/vec[E;F] = b_i    ==
  data: E input; vec_EF output; F input
function vec_EF = fcn(E,F)
[Ec,Er] = size(E);
[Fc,Fr] = size(F);
vec_EF = reshape([E;F],Ec*Er+Fc*Fr,1);
end

== matlab function Adaptive_Distributed_Observer/Adaptive Output Regulator 4/Regulator/Create Q ==
  data: Q_T output size=[3*n,3*n]; Q output size=[3*n,3*n]; S input; B input; A input
function [Q_T,Q]= fcn(S,B,A)
[Sc,Sr]=size(S);
I_ni = [eye(2) zeros(2,1);zeros(1,3)];
I_q = eye(Sc);
sysmatrix = [A B;1 0 0];

Q = kron(S.',I_ni)-kron(I_q,sysmatrix);
Q_T = Q.';
end

== matlab function Adaptive_Distributed_Observer/Adaptive Output Regulator 4/Regulator/Kx ==
  data: B input; A input; Kx output; p input
function Kx = fcn(B,A,p)

coder.extrinsic('place')
Kx = zeros(1,2);
Kx = place(A,-B,p);

== matlab function Adaptive_Distributed_Observer/Adaptive Output Regulator 4/Regulator/inverse reshape ==
  data: zeta input; X output; U output
function [X,U] = fcn(zeta)
n = 4;
tmp = reshape(zeta,3,n);
X = tmp(1:2,1:n);
U = tmp(3,:);
end

== matlab function Adaptive_Distributed_Observer/Adaptive Output Regulator 4/Regulator/vec[E;F] = b_i    ==
  data: E input; vec_EF output; F input
function vec_EF = fcn(E,F)
[Ec,Er] = size(E);
[Fc,Fr] = size(F);
vec_EF = reshape([E;F],Ec*Er+Fc*Fr,1);
end
